simulink model "RLC"  (Simulink 4.00)
settings: Solver=ode23tb  StartTime=0.0  StopTime=0.1  RelTol=1e-3
InitFcn:
  | powericon('psbinitsys',bdroot);
libraries: powerlib2 x8
settings Model: LastModifiedBy=ieao

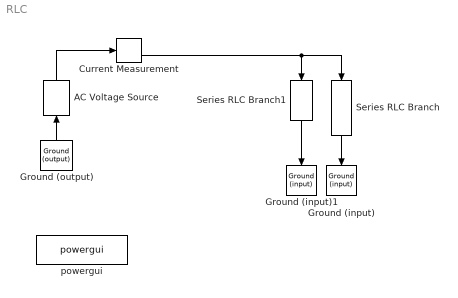
== system RLC ==
  AC Voltage Source : powerlib2/Electrical Sources/AC Voltage Source  Tag=PoWeRsYsTeMbLoCk  Orientation=up  A=10  P=0  F=100  stime=0  mesure=None  PSBOutputType=1
  Current Measurement : powerlib2/Measurements/Current Measurement  Tag=PoWeRsYsTeMmEaSuReMeNt  PSBOutputType=01  PSBequivalent=1
  Ground (input) : powerlib2/Connectors/Ground (input)  Tag=PoWeRsYsTeMbLoCk  Orientation=down
  Ground (input)1 : powerlib2/Connectors/Ground (input)  Tag=PoWeRsYsTeMbLoCk  Orientation=down
  Ground (output) : powerlib2/Connectors/Ground (output)  Tag=PoWeRsYsTeMbLoCk  Orientation=up  PSBOutputType=1
  Series RLC Branch : powerlib2/Elements/Series RLC Branch  Tag=PoWeRsYsTeMbLoCk  Orientation=down  a=20  b=1e-02  c=inf  mesure=None  PSBOutputType=1
  Series RLC Branch1 : powerlib2/Elements/Series RLC Branch  Tag=PoWeRsYsTeMbLoCk  Orientation=down  a=0.01  b=0  c=1e-05  mesure=None  PSBOutputType=1
  powergui : powerlib2/powergui  matfilesaved=off  Frange=logspace(0,3,50)  Ylog=off  Xlog=off  save=off  variable=ZData  display=off  Ts=0  methode=off  frequency=60  echomessages=off
  wires:
  AC Voltage Source/1 -> Current Measurement/1
  Current Measurement/2 -> Series RLC Branch1/1, Series RLC Branch/1
  Ground (output)/1 -> AC Voltage Source/1
  Series RLC Branch/1 -> Ground (input)/1
  Series RLC Branch1/1 -> Ground (input)1/1
